simulink subsystem "sensor"  (R2024b)
settings: Solver=VariableStepAuto  StartTime=0.0  StopTime=10.0  RelTol=1e-3
settings Model: Creator=Asus  LastModifiedBy=Asus

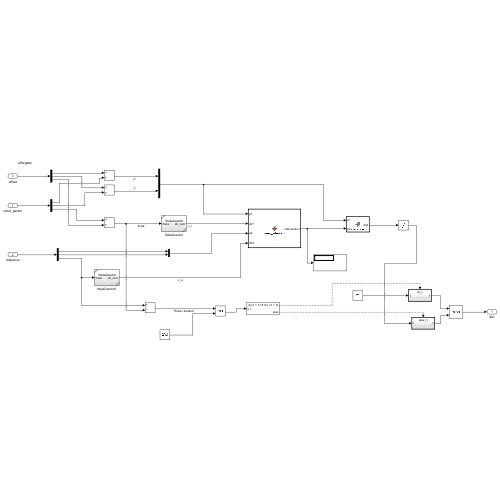
[thumbnail: Simulink's stored preview of the top-level diagram]
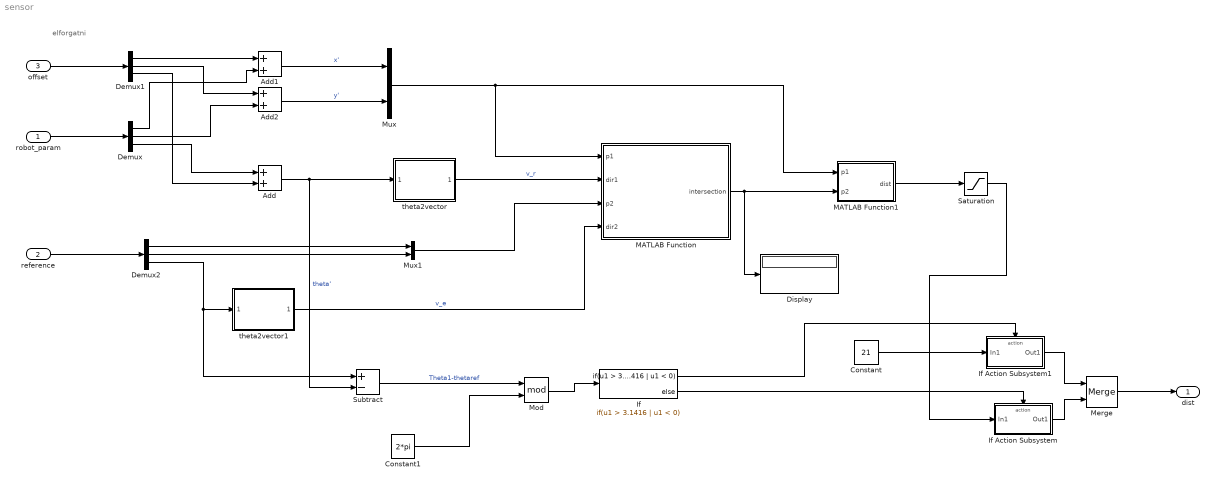
== system sensor ==
  note: elforgatni
  robot_param : Inport
  reference : Inport  Port=2
  offset : Inport  Port=3
  Add : Sum
  Add1 : Sum
  Add2 : Sum
  Constant : Constant  Value=21
  Constant1 : Constant  Value=2*pi
  Demux : Demux  Outputs=3
  Demux1 : Demux  Outputs=3
  Demux2 : Demux  Outputs=3
  Display : Display
  If : If  IfExpression=u1 > 3.1416 | u1 < 0
  If Action Subsystem : Subsystem  TreatAsAtomicUnit=on
  If Action Subsystem1 : Subsystem  TreatAsAtomicUnit=on
  MATLAB Function : MATLAB Function  TreatAsAtomicUnit=on
  MATLAB Function1 : MATLAB Function  TreatAsAtomicUnit=on
  Merge : Merge
  Mod : Math  Operator=mod
  Mux : Mux  Inputs=2
  Mux1 : Mux  Inputs=2
  Saturation : Saturate  UpperLimit=20  LowerLimit=0
  Subtract : Sum  Inputs=+-
  theta2vector : Subsystem  ReferencedSubsystem=theta2vector
  theta2vector1 : Subsystem  ReferencedSubsystem=theta2vector
  dist : Outport
  wires:
  robot_param/1 -> Demux/1
  Demux/3 -> Add/1
  Add/1 -> Subtract/2, theta2vector/1  "theta'"
  offset/1 -> Demux1/1
  Demux1/1 -> Add1/1
  Demux1/2 -> Add2/1
  Demux/1 -> Add1/2
  Demux/2 -> Add2/2
  Add2/1 -> Mux/2  "y'"
  Add1/1 -> Mux/1  "x'"
  reference/1 -> Demux2/1
  theta2vector/1 -> MATLAB Function/2(dir1)  "v_r"
  theta2vector1/1 -> MATLAB Function/4(dir2)  "v_e"
  Demux2/3 -> Subtract/1, theta2vector1/1
  Mux/1 -> MATLAB Function/1(p1), MATLAB Function1/1(p1)
  Mux1/1 -> MATLAB Function/3(p2)
  Demux2/1 -> Mux1/1
  Demux2/2 -> Mux1/2
  MATLAB Function1/1(dist) -> Saturation/1
  MATLAB Function/1(intersection) -> MATLAB Function1/2(p2), Display/1
  Demux1/3 -> Add/2
  Saturation/1 -> If Action Subsystem/1(In1)
  Subtract/1 -> Mod/1  "Theta1-thetaref"
  If/2 -> If Action Subsystem/Action
  Merge/1 -> dist/1
  If Action Subsystem/1(Out1) -> Merge/2
  If Action Subsystem1/1(Out1) -> Merge/1
  If/1 -> If Action Subsystem1/Action
  Constant/1 -> If Action Subsystem1/1(In1)
  Mod/1 -> If/1
  Constant1/1 -> Mod/2

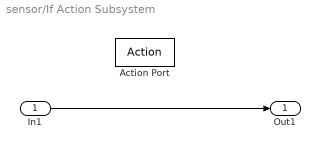
== system sensor/If Action Subsystem ==
  In1 : Inport
  Action Port : ActionPort  ActionPortLabel=else
  Out1 : Outport
  wires:
  In1/1 -> Out1/1

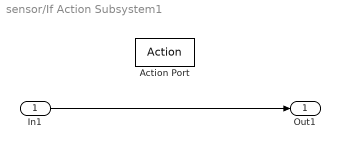
== system sensor/If Action Subsystem1 ==
  In1 : Inport
  Action Port : ActionPort  ActionPortLabel=if(u1 > 3.1416 | u1 < 0)
  Out1 : Outport
  wires:
  In1/1 -> Out1/1

== matlab function sensor/MATLAB Function1 ==
  data: p1 input; dist output; p2 input
function dist = distance(p1, p2)

dist = norm(p1-p2);

== matlab function sensor/MATLAB Function ==
  data: p1 input; intersection output; dir1 input; p2 input; dir2 input
function intersection = lines_intersect(p1, dir1, p2, dir2)
%inicialisation:    
    arguments(Input)
        p1 (2,1) double 
        dir1 (2,1) double
        p2 (2,1) double
        dir2 (2,1) double
    end
    arguments(Output)
        intersection (2, 1) double
    end
    line1 = zeros(1,3);
    line2 = zeros(1,3);
    intersection = zeros(2,1);
%LINE_INTERSECT Summary of this function goes here
%   Detailed explanation goes here
    
    % source: https://en.wikipedia.org/wiki/Line%E2%80%93line_intersection#Using_homogeneous_coordinates
    
    % normal vectors
    n1 = [dir1(2), -dir1(1)];
    n2 = [dir2(2), -dir2(1)];
    
    % line description with a*x + b*y + c = 0
    % (n_1*x + n_2*y = n_1*x0 + n_2*y0
    line1 = [n1(1), n1(2), -dot(p1, n1)];
    line2 = [n2(1), n2(2), -dot(p2, n2)];
    
    % intersection in homogeneous coordinates
    intersection_hom = cross(line1, line2);
    
    % convert the homogeneous coordinates to cartesian
    if(abs(intersection_hom(3)) < 1e-6)
        intersection = [10e5 10e5];
    else
        intersection = [intersection_hom(1)/intersection_hom(3), intersection_hom(2)/intersection_hom(3)];
    end
end
